simulink model "yalinySatSim"  (R2015b)
settings: Solver=ode45  StartTime=0.0  StopTime=100  RelTol=1e-3
values from neighbouring files (symbols this model uses):
  orbData =     [orbitData.mat]
undefined symbols (not defined in the file or in its folder): e0_0, e1_0, e2_0, e3_0, params
libraries: aerolibutil x16, vrlib x16, satellite_control_lib x11, aerolibtransform2 x3, aerolib6dofsys x2, simulink_extras x1
settings Model: Creator=DNikolaev  LastModifiedBy=DNikolaev

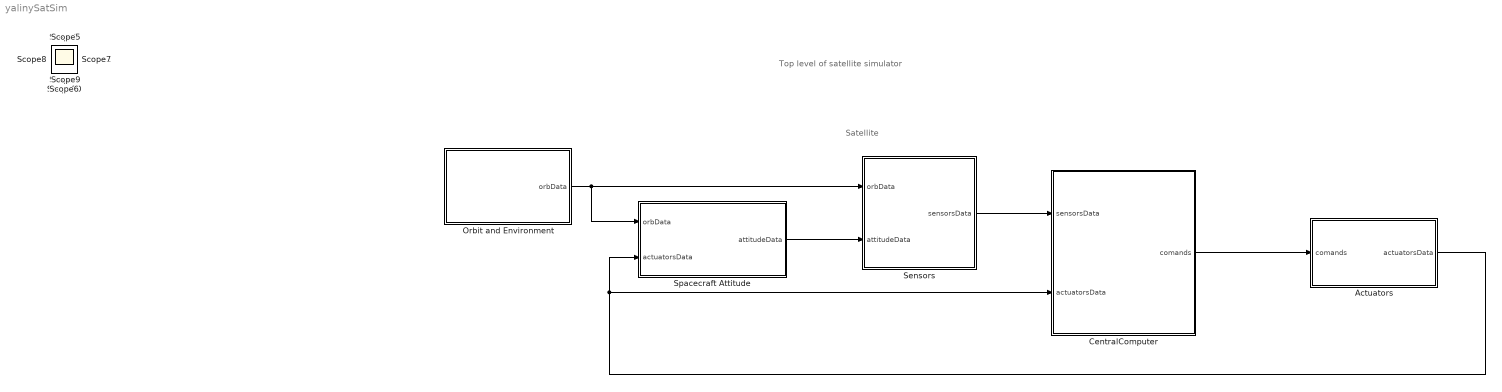
== system yalinySatSim ==
  note: Satellite
  note: Top level of satellite simulator
  Actuators : Subsystem
  CentralComputer : Subsystem
  Orbit and Environment : Subsystem
  Sensors : Subsystem
  Spacecraft Attitude : Subsystem
  Scope{,1..10} (11 alike) : Scope
  wires:
  Sensors/1(sensorsData) -> CentralComputer/1(sensorsData)
  Actuators/1(actuatorsData) -> CentralComputer/2(actuatorsData), Spacecraft Attitude/2(actuatorsData)
  CentralComputer/1(comands) -> Actuators/1(comands)
  Orbit and Environment/1(orbData) -> Spacecraft Attitude/1(orbData), Sensors/1(orbData)
  Spacecraft Attitude/1(attitudeData) -> Sensors/2(attitudeData)

== system yalinySatSim/Actuators ==
  comands : Inport
  Bus Creator : BusCreator  Inputs=3
  Bus Selector4 : BusSelector  OutputSignals=Urw,Umagn
  Constant2 : Constant  Value=[0 0 0]
  Magnetic Coils : satellite_control_lib/Actuators/Magnetic Coils  MagnMomentMax=params.MagnMomentMax
  Manual Switch : ManualSwitch
  Reaction Wheels 4-pyramid configuration : satellite_control_lib/Actuators/Reaction Wheels 4-pyramid configuration  VariantControl=Variant  Hrwmax=params.Hrwmax  Trwmax=params.Trwmax  delta=params.rwdelta  gamma=params.rwgamma  sampleTime=0.1
  actuatorsData : Outport
  wires:
  comands/1 -> Bus Selector4/1
  Bus Creator/1 -> actuatorsData/1
  Magnetic Coils/1 -> Bus Creator/3  "L"
  Bus Selector4/1 -> Manual Switch/1  "<Urw>"
  Manual Switch/1 -> Reaction Wheels 4-pyramid configuration/1
  Constant2/1 -> Manual Switch/2
  Reaction Wheels 4-pyramid configuration/1 -> Bus Creator/1  "Trw_p"
  Reaction Wheels 4-pyramid configuration/2 -> Bus Creator/2  "Hrw_p"
  Bus Selector4/2 -> Magnetic Coils/1  "<Umagn >"

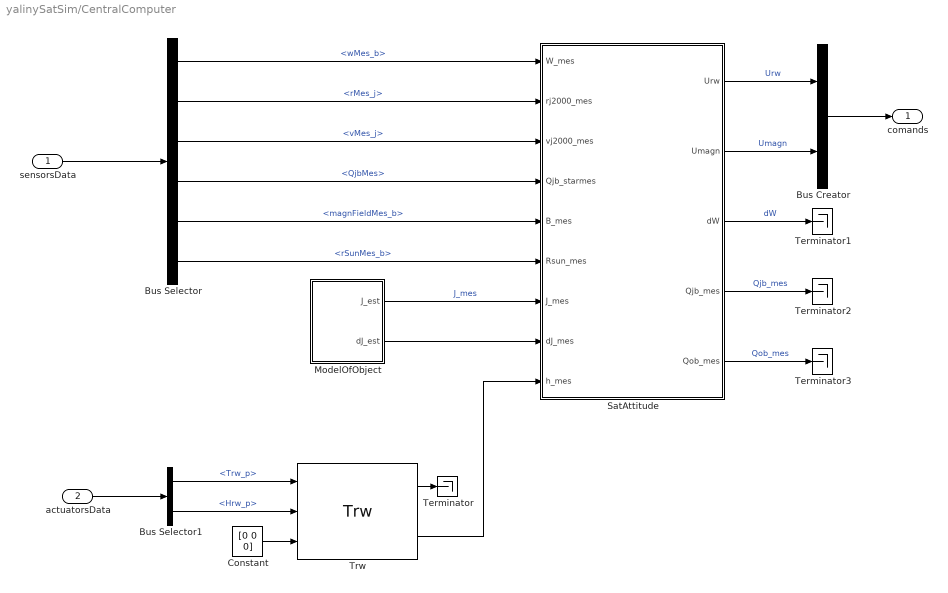
== system yalinySatSim/CentralComputer ==
  sensorsData : Inport
  actuatorsData : Inport  Port=2
  Bus Creator : BusCreator  Inputs=2
  Bus Selector : BusSelector  OutputSignals=wMes_b,rMes_j,vMes_j,QjbMes,magnFieldMes_b,rSunMes_b
  Bus Selector1 : BusSelector  OutputSignals=Trw_p,Hrw_p
  Constant : Constant  Value=[0 0 0]
  ModelOfObject : Subsystem
  SatAttitude : Subsystem
  Terminator{,1..3} (4 alike) : Terminator
  Trw : satellite_control_lib/Torques/Trw  delta=params.rwdelta  gamma=params.rwgamma
  comands : Outport
  wires:
  sensorsData/1 -> Bus Selector/1
  Bus Creator/1 -> comands/1
  ModelOfObject/1(J_est) -> SatAttitude/7(J_mes)  "J_mes"
  SatAttitude/1(Urw) -> Bus Creator/1  "Urw"
  ModelOfObject/2(dJ_est) -> SatAttitude/8(dJ_mes)
  Trw/2 -> SatAttitude/9(h_mes)
  actuatorsData/1 -> Bus Selector1/1
  Bus Selector/2 -> SatAttitude/2(rj2000_mes)  "<rMes_j>"
  Bus Selector/3 -> SatAttitude/3(vj2000_mes)  "<vMes_j>"
  Bus Selector/6 -> SatAttitude/6(Rsun_mes)  "<rSunMes_b>"
  Bus Selector/5 -> SatAttitude/5(B_mes)  "<magnFieldMes_b>"
  Bus Selector/1 -> SatAttitude/1(W_mes)  "<wMes_b>"
  Bus Selector/4 -> SatAttitude/4(Qjb_starmes)  "<QjbMes>"
  Bus Selector1/1 -> Trw/1  "<Trw_p>"
  Bus Selector1/2 -> Trw/2  "<Hrw_p>"
  Trw/1 -> Terminator/1
  Constant/1 -> Trw/3
  SatAttitude/3(dW) -> Terminator1/1  "dW"
  SatAttitude/4(Qjb_mes) -> Terminator2/1  "Qjb_mes"
  SatAttitude/5(Qob_mes) -> Terminator3/1  "Qob_mes"
  SatAttitude/2("Umagn ") -> Bus Creator/2  "Umagn"

== system yalinySatSim/Orbit and Environment ==
  Precomputed Data : FromWorkspace  VariableName=inOrbData  OutDataTypeStr=Bus: orbBus  SampleTime=0  OutputAfterFinalValue=Holding final value
  orbData : Outport
  wires:
  Precomputed Data/1 -> orbData/1

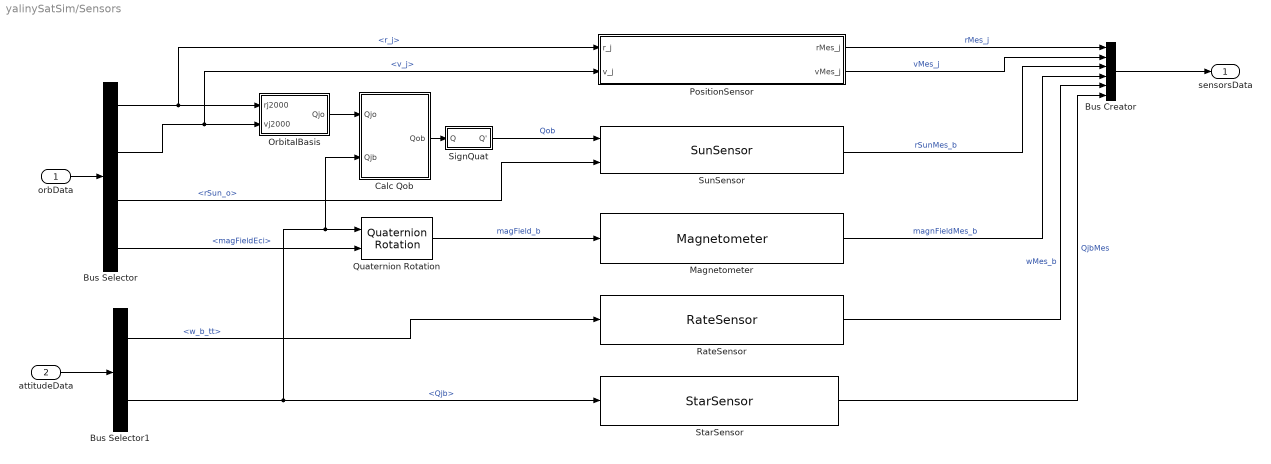
== system yalinySatSim/Sensors ==
  orbData : Inport
  attitudeData : Inport  Port=2
  Bus Creator : BusCreator  Inputs=6
  Bus Selector : BusSelector  OutputSignals=r_j,v_j,rSun_o,magFieldEci
  Bus Selector1 : BusSelector  OutputSignals=w_b_tt,Qjb
  Calc Qob : Subsystem
  Magnetometer : satellite_control_lib/Sensors/Magnetometer  S=[0 0 0;0 0 0;0 0 0]  bias=0  sigma2=0  seed=0  outputSampleTime=0.1
  OrbitalBasis : Subsystem
  PositionSensor : Subsystem
  Quaternion Rotation : aerolibutil/Quaternion Rotation
  RateSensor : satellite_control_lib/Sensors/RateSensor  S=[0 0 0;0 0 0;0 0 0]  sigma2_b=0  seed_b=[0 0 0]  sigma2_n=1e-6  seed=[0 0 0]  rateSensorSamleTime=0.1
  SignQuat : Subsystem
  StarSensor : satellite_control_lib/Sensors/StarSensor  sigma2=[0 0 0]  seed=[0 0 0]  outputSamleTime=0.1
  SunSensor : satellite_control_lib/Sensors/SunSensor  sigma2=[0 0 0]  seed=[0 0 0]  outputSampleTime=0.1
  sensorsData : Outport
  wires:
  orbData/1 -> Bus Selector/1
  attitudeData/1 -> Bus Selector1/1
  Bus Selector/1 -> PositionSensor/1(r_j), OrbitalBasis/1(rj2000)  "<r_j>"
  Bus Selector/2 -> PositionSensor/2(v_j), OrbitalBasis/2(vj2000)  "<v_j>"
  Bus Selector/3 -> SunSensor/2  "<rSun_o>"
  Bus Selector/4 -> Quaternion Rotation/2  "<magFieldEci>"
  Bus Selector1/2 -> Quaternion Rotation/1, Calc Qob/2(Qjb), StarSensor/1  "<Qjb>"
  Bus Selector1/1 -> RateSensor/1  "<w_b_tt>"
  Bus Creator/1 -> sensorsData/1
  RateSensor/1 -> Bus Creator/5  "wMes_b"
  Quaternion Rotation/1 -> Magnetometer/1  "magField_b"
  Magnetometer/1 -> Bus Creator/4  "magnFieldMes_b"
  Calc Qob/1(Qob) -> SignQuat/1(Q)
  OrbitalBasis/1(Qjo) -> Calc Qob/1(Qjo)
  SignQuat/1(Q') -> SunSensor/1  "Qob"
  SunSensor/1 -> Bus Creator/3  "rSunMes_b"
  PositionSensor/1(rMes_j) -> Bus Creator/1  "rMes_j"
  PositionSensor/2(vMes_j) -> Bus Creator/2  "vMes_j"
  StarSensor/1 -> Bus Creator/6  "QjbMes"

== system yalinySatSim/Spacecraft Attitude ==
  orbData : Inport
  actuatorsData : Inport  Port=2
  Bus Creator : BusCreator  Inputs=2
  Inertia : Subsystem
  Spacecraft Dynamics : Subsystem
  Torques : Subsystem
  attitudeData : Outport
  wires:
  Torques/1(T) -> Spacecraft Dynamics/1(T)
  Inertia/1(Inertia) -> Spacecraft Dynamics/2(Inertia), Torques/5(Inertia)
  Inertia/2(dInertia) -> Spacecraft Dynamics/3(dInertia)
  Spacecraft Dynamics/2(w_b) -> Bus Creator/2, Torques/2(w_b)  "w_b_tt"
  Bus Creator/1 -> attitudeData/1
  orbData/1 -> Torques/3(orbData)
  actuatorsData/1 -> Torques/4(actuatorsData)
  Spacecraft Dynamics/1(Qjb) -> Torques/1(Qjb), Bus Creator/1  "Qjb"

== system yalinySatSim/CentralComputer/ModelOfObject ==
  ChangeMe1 : Constant  Value=zeros(3)
  ChangeMe2 : Constant  Value=1000*eye(3)
  J_est : Outport
  dJ_est : Outport  Port=2
  wires:
  ChangeMe1/1 -> dJ_est/1
  ChangeMe2/1 -> J_est/1

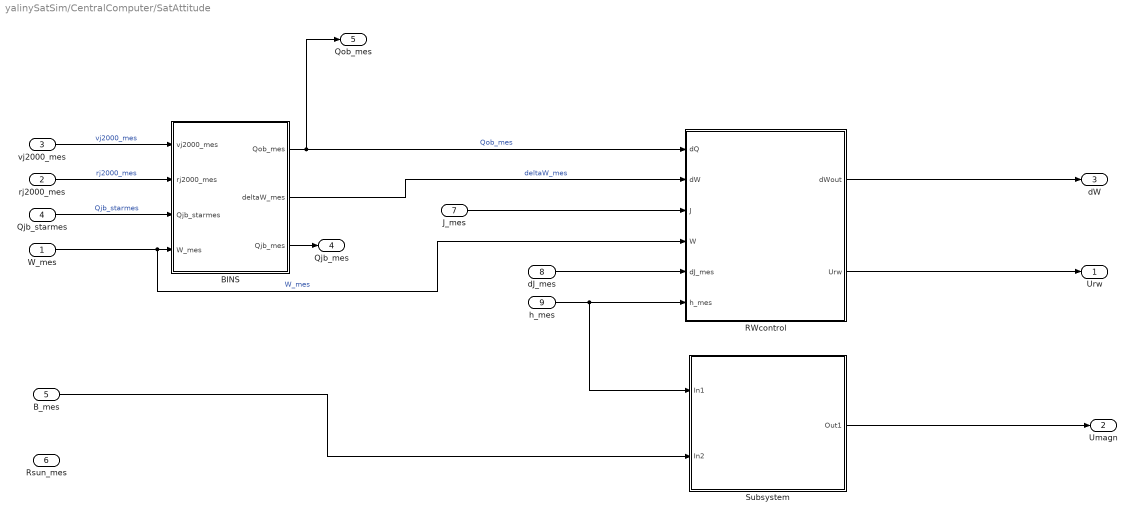
== system yalinySatSim/CentralComputer/SatAttitude ==
  W_mes : Inport
  rj2000_mes : Inport  Port=2
  vj2000_mes : Inport  Port=3
  Qjb_starmes : Inport  Port=4
  B_mes : Inport  Port=5
  Rsun_mes : Inport  Port=6
  J_mes : Inport  Port=7
  dJ_mes : Inport  Port=8
  h_mes : Inport  Port=9
  BINS : Subsystem
  RWcontrol : Subsystem
  Subsystem : Subsystem
  Urw : Outport
  "Umagn " : Outport  Port=2
  dW : Outport  Port=3
  Qjb_mes : Outport  Port=4
  Qob_mes : Outport  Port=5
  wires:
  vj2000_mes/1 -> BINS/1(vj2000_mes)  "vj2000_mes"
  rj2000_mes/1 -> BINS/2(rj2000_mes)  "rj2000_mes"
  Qjb_starmes/1 -> BINS/3(Qjb_starmes)  "Qjb_starmes"
  W_mes/1 -> RWcontrol/4(W), BINS/4(W_mes)  "W_mes"
  BINS/1(Qob_mes) -> Qob_mes/1, RWcontrol/1(dQ)  "Qob_mes"
  BINS/3(Qjb_mes) -> Qjb_mes/1
  BINS/2(deltaW_mes) -> RWcontrol/2(dW)  "deltaW_mes"
  J_mes/1 -> RWcontrol/3(J)
  dJ_mes/1 -> RWcontrol/5(dJ_mes)
  h_mes/1 -> Subsystem/1(In1), RWcontrol/6(h_mes)
  RWcontrol/1(dWout) -> dW/1
  RWcontrol/2(Urw) -> Urw/1
  B_mes/1 -> Subsystem/2(In2)
  Subsystem/1(Out1) -> "Umagn "/1

== system yalinySatSim/Sensors/Calc Qob ==
  Qjo : Inport
  Qjb : Inport  Port=2
  Quaternion Inverse : aerolibutil/Quaternion Inverse
  Quaternion Multiplication : aerolibutil/Quaternion Multiplication
  Qob : Outport
  wires:
  Qjb/1 -> Quaternion Multiplication/2  "Qjb"
  Qjo/1 -> Quaternion Inverse/1  "Qjo"
  Quaternion Inverse/1 -> Quaternion Multiplication/1
  Quaternion Multiplication/1 -> Qob/1

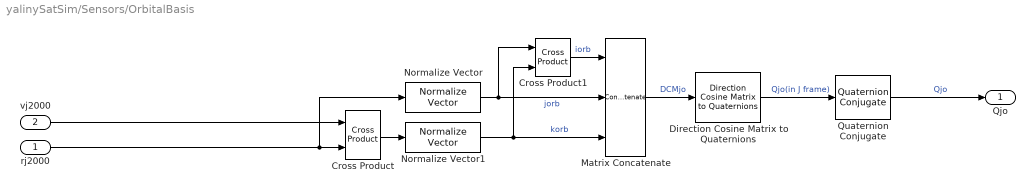
== system yalinySatSim/Sensors/OrbitalBasis ==
  rj2000 : Inport
  vj2000 : Inport  Port=2
  Cross Product : vrlib/Utilities/Cross Product
  Cross Product1 : vrlib/Utilities/Cross Product
  Direction Cosine Matrix to Quaternions : aerolibtransform2/Direction Cosine Matrix  to Quaternions
  Matrix Concatenate : Concatenate  NumInputs=3  Mode=Multidimensional array  ConcatenateDimension=2
  Normalize Vector : vrlib/Utilities/Normalize Vector  maxzero=0.00001
  Normalize Vector1 : vrlib/Utilities/Normalize Vector  maxzero=0.00001
  Quaternion Conjugate : aerolibutil/Quaternion Conjugate
  Qjo : Outport
  wires:
  Quaternion Conjugate/1 -> Qjo/1  "Qjo"
  Cross Product/1 -> Normalize Vector1/1
  Normalize Vector1/1 -> Cross Product1/2, Matrix Concatenate/3  "korb"
  Direction Cosine Matrix to Quaternions/1 -> Quaternion Conjugate/1  "Qjo(in J frame)"
  vj2000/1 -> Cross Product/1
  rj2000/1 -> Cross Product/2, Normalize Vector/1
  Matrix Concatenate/1 -> Direction Cosine Matrix to Quaternions/1  "DCMjo"
  Normalize Vector/1 -> Cross Product1/1, Matrix Concatenate/2  "jorb"
  Cross Product1/1 -> Matrix Concatenate/1  "iorb"

== system yalinySatSim/Sensors/PositionSensor ==
  r_j : Inport
  v_j : Inport  Port=2
  Zero-Order Hold : ZeroOrderHold  SampleTime=0.1
  Zero-Order Hold1 : ZeroOrderHold  SampleTime=0.1
  rMes_j : Outport
  vMes_j : Outport  Port=2
  wires:
  Zero-Order Hold/1 -> rMes_j/1
  Zero-Order Hold1/1 -> vMes_j/1
  r_j/1 -> Zero-Order Hold/1
  v_j/1 -> Zero-Order Hold1/1

== system yalinySatSim/Sensors/SignQuat ==
  Q : Inport
  Product : Product
  Selector2 : Selector  InputPortWidth=4  IndexOptions=Index vector (dialog)  Indices=[1]  OutputSizes=1
  Sign : Signum
  Q' : Outport
  wires:
  Q/1 -> Product/2, Selector2/1
  Product/1 -> Q'/1
  Sign/1 -> Product/1
  Selector2/1 -> Sign/1

== system yalinySatSim/Spacecraft Attitude/Inertia ==
  bodysAttitude : Inport
  Constant : Constant  Value=1000*eye(3)
  Constant1 : Constant  Value=zeros(3)
  Inertia : Outport
  dInertia : Outport  Port=2
  wires:
  Constant1/1 -> dInertia/1
  Constant/1 -> Inertia/1

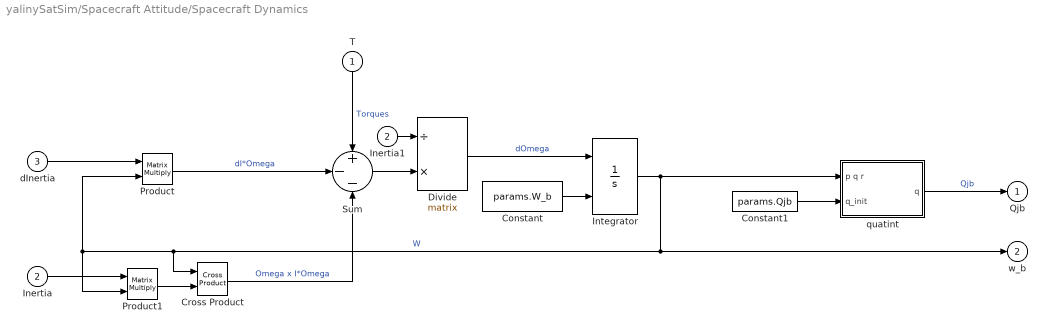
== system yalinySatSim/Spacecraft Attitude/Spacecraft Dynamics ==
  T : Inport
  Inertia : Inport  Port=2
  dInertia : Inport  Port=3
  Constant : Constant  Value=params.W_b
  Constant1 : Constant  Value=params.Qjb
  Cross Product : vrlib/Utilities/Cross Product
  Divide : Product  Inputs=/*  Multiplication=Matrix(*)
  Inertia1 : InportShadow  Port=2
  Integrator : Integrator  InitialConditionSource=external
  Product : Product  Multiplication=Matrix(*)
  Product1 : Product  Multiplication=Matrix(*)
  Sum : Sum  Inputs=+--
  quatint : Subsystem
  Qjb : Outport
  w_b : Outport  Port=2
  wires:
  Sum/1 -> Divide/2
  Inertia1/1 -> Divide/1
  Divide/1 -> Integrator/1  "dOmega"
  Constant/1 -> Integrator/2
  Product/1 -> Sum/2  "dI*Omega"
  dInertia/1 -> Product/1
  Constant1/1 -> quatint/2(q_init)
  quatint/1(q) -> Qjb/1  "Qjb"
  Inertia/1 -> Product1/1
  Product1/1 -> Cross Product/2
  Cross Product/1 -> Sum/3  "Omega x I*Omega"
  Integrator/1 -> quatint/1(p q r), Cross Product/1, Product/2, Product1/2, w_b/1  "W"
  T/1 -> Sum/1  "Torques"

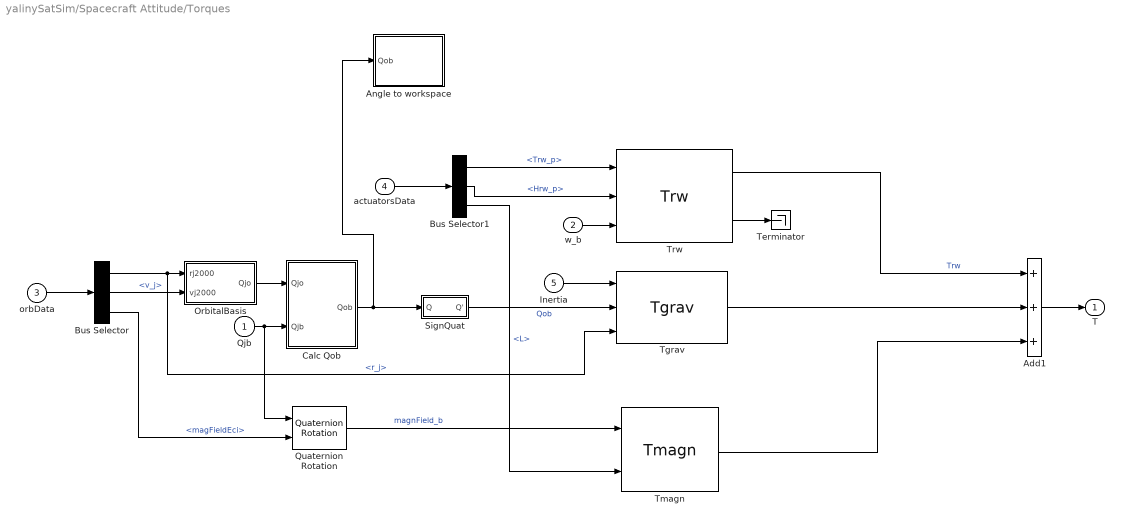
== system yalinySatSim/Spacecraft Attitude/Torques ==
  Qjb : Inport
  w_b : Inport  Port=2
  orbData : Inport  Port=3
  actuatorsData : Inport  Port=4
  Inertia : Inport  Port=5
  Add1 : Sum  Inputs=3
  Angle to workspace : Subsystem
  Bus Selector : BusSelector  OutputSignals=r_j,v_j,magFieldEci
  Bus Selector1 : BusSelector  OutputSignals=Trw_p,Hrw_p,L
  Calc Qob : Subsystem
  OrbitalBasis : Subsystem
  Quaternion Rotation : aerolibutil/Quaternion Rotation
  SignQuat : Subsystem
  Terminator : Terminator
  Tgrav : satellite_control_lib/Torques/Tgrav
  Tmagn : satellite_control_lib/Torques/Tmagn
  Trw : satellite_control_lib/Torques/Trw  delta=params.rwdelta  gamma=params.rwgamma
  T : Outport
  wires:
  Add1/1 -> T/1
  Trw/1 -> Add1/1  "Trw"
  Tgrav/1 -> Add1/2
  orbData/1 -> Bus Selector/1
  actuatorsData/1 -> Bus Selector1/1
  SignQuat/1(Q') -> Tgrav/2  "Qob"
  Bus Selector/1 -> Tgrav/3, OrbitalBasis/1(rj2000)  "<r_j>"
  Bus Selector/2 -> OrbitalBasis/2(vj2000)  "<v_j>"
  OrbitalBasis/1(Qjo) -> Calc Qob/1(Qjo)
  Qjb/1 -> Quaternion Rotation/1, Calc Qob/2(Qjb)
  Inertia/1 -> Tgrav/1
  w_b/1 -> Trw/3
  Bus Selector1/2 -> Trw/2  "<Hrw_p>"
  Bus Selector1/1 -> Trw/1  "<Trw_p>"
  Trw/2 -> Terminator/1
  Tmagn/1 -> Add1/3
  Bus Selector/3 -> Quaternion Rotation/2  "<magFieldEci>"
  Quaternion Rotation/1 -> Tmagn/1  "magnField_b"
  Bus Selector1/3 -> Tmagn/2  "<L>"
  Calc Qob/1(Qob) -> Angle to workspace/1(Qob), SignQuat/1(Q)

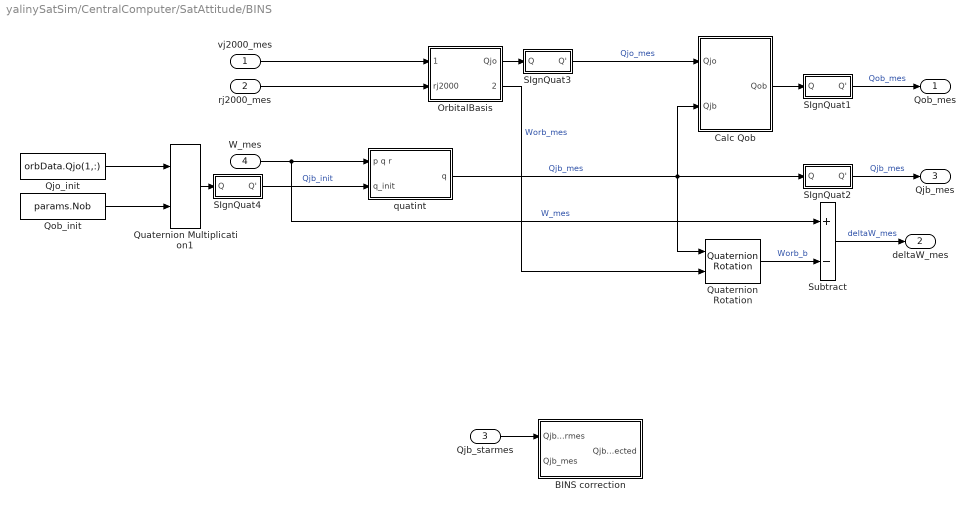
== system yalinySatSim/CentralComputer/SatAttitude/BINS ==
  vj2000_mes : Inport
  rj2000_mes : Inport  Port=2
  Qjb_starmes : Inport  Port=3
  W_mes : Inport  Port=4
  BINS correction : Subsystem
  Calc Qob : Subsystem
  OrbitalBasis : Subsystem
  Qjo_init : Constant  Value=orbData.Qjo(1,:)
  Qob_init : Constant  Value=params.Nob
  Quaternion Multiplication1 : aerolibutil/Quaternion Multiplication
  Quaternion Rotation : aerolibutil/Quaternion Rotation
  SIgnQuat1 : Subsystem
  SIgnQuat2 : Subsystem
  SIgnQuat3 : Subsystem
  SIgnQuat4 : Subsystem
  Subtract : Sum  Inputs=+-
  quatint : Subsystem  mask{k_quat=1}
      mask prompts: k_quat "Quaternion normalization gain"
  Qob_mes : Outport
  deltaW_mes : Outport  Port=2
  Qjb_mes : Outport  Port=3
  wires:
  Qjb_starmes/1 -> BINS correction/1(Qjb_starmes)
  quatint/1(q) -> SIgnQuat2/1(Q), Calc Qob/2(Qjb), Quaternion Rotation/1  "Qjb_mes"
  Calc Qob/1(Qob) -> SIgnQuat1/1(Q)
  rj2000_mes/1 -> OrbitalBasis/2(rj2000)
  vj2000_mes/1 -> OrbitalBasis/1(vj2000)
  OrbitalBasis/1(Qjo) -> SIgnQuat3/1(Q)
  OrbitalBasis/2(Worb_j) -> Quaternion Rotation/2  "Worb_mes"
  W_mes/1 -> Subtract/1, quatint/1(p q r)  "W_mes"
  Subtract/1 -> deltaW_mes/1  "deltaW_mes"
  Qjo_init/1 -> Quaternion Multiplication1/1
  Qob_init/1 -> Quaternion Multiplication1/2
  Quaternion Multiplication1/1 -> SIgnQuat4/1(Q)
  Quaternion Rotation/1 -> Subtract/2  "Worb_b"
  SIgnQuat1/1(Q') -> Qob_mes/1  "Qob_mes"
  SIgnQuat2/1(Q') -> Qjb_mes/1  "Qjb_mes"
  SIgnQuat3/1(Q') -> Calc Qob/1(Qjo)  "Qjo_mes"
  SIgnQuat4/1(Q') -> quatint/2(q_init)  "Qjb_init"

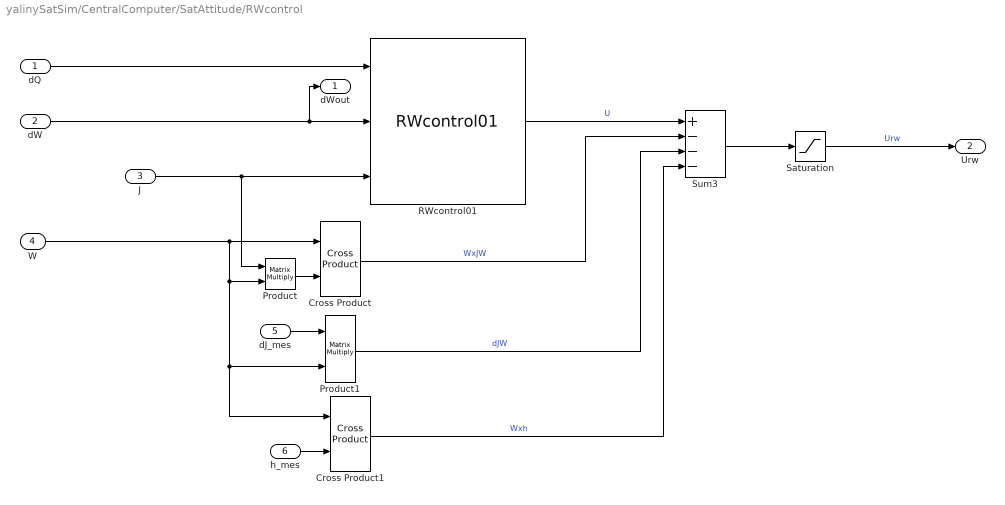
== system yalinySatSim/CentralComputer/SatAttitude/RWcontrol ==
  dQ : Inport
  dW : Inport  Port=2
  J : Inport  Port=3
  W : Inport  Port=4
  dJ_mes : Inport  Port=5
  h_mes : Inport  Port=6
  Cross Product : vrlib/Utilities/Cross Product
  Cross Product1 : vrlib/Utilities/Cross Product
  Product : Product  Multiplication=Matrix(*)
  Product1 : Product  Multiplication=Matrix(*)
  RWcontrol01 : satellite_control_lib/RWcontrol01  Kq=params.K1acs  Kw=params.K2acs
  Saturation : Saturate  UpperLimit=0.1  LowerLimit=-0.1
  Sum3 : Sum  Inputs=+---
  dWout : Outport
  Urw : Outport  Port=2
  wires:
  W/1 -> Product/2, Product1/2, Cross Product1/1, Cross Product/1
  dQ/1 -> RWcontrol01/1
  RWcontrol01/1 -> Sum3/1  "U"
  J/1 -> Product/1, RWcontrol01/3
  dW/1 -> dWout/1, RWcontrol01/2
  Product/1 -> Cross Product/2
  Cross Product/1 -> Sum3/2  "WxJW"
  Product1/1 -> Sum3/3  "dJW"
  Cross Product1/1 -> Sum3/4  "Wxh"
  h_mes/1 -> Cross Product1/2
  dJ_mes/1 -> Product1/1
  Saturation/1 -> Urw/1  "Urw"
  Sum3/1 -> Saturation/1

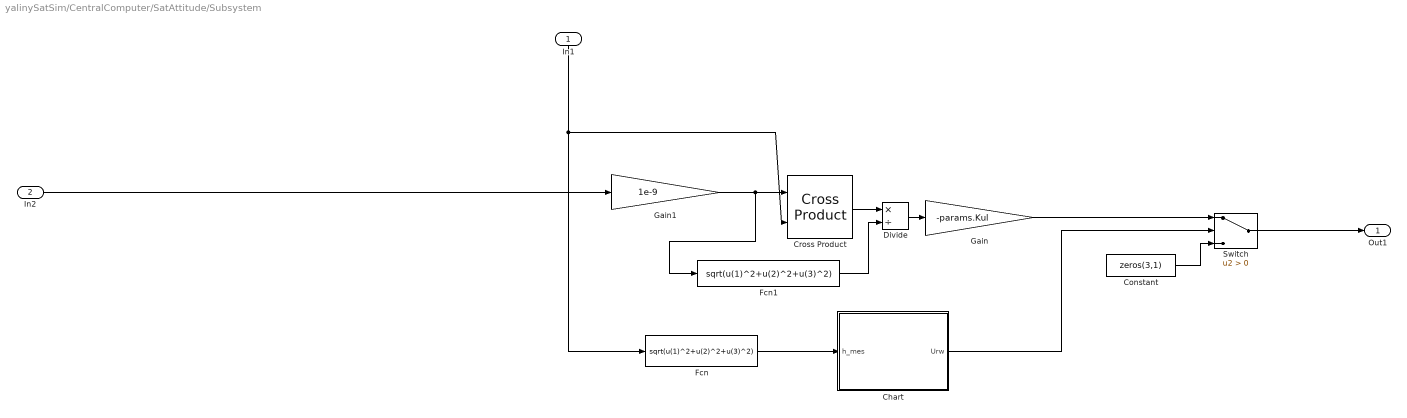
== system yalinySatSim/CentralComputer/SatAttitude/Subsystem ==
  In1 : Inport
  In2 : Inport  Port=2
  Chart : Stateflow chart  TreatAsAtomicUnit=on
  Constant : Constant  Value=zeros(3,1)
  Cross Product : vrlib/Utilities/Cross Product
  Divide : Product  Inputs=*/
  Fcn : Fcn  Expr=sqrt(u(1)^2+u(2)^2+u(3)^2)
  Fcn1 : Fcn  Expr=sqrt(u(1)^2+u(2)^2+u(3)^2)
  Gain : Gain  Gain=-params.Kul
  Gain1 : Gain  Gain=1e-9
  Switch : Switch  Criteria=u2 > Threshold
  Out1 : Outport
  wires:
  In1/1 -> Cross Product/2, Fcn/1
  In2/1 -> Gain1/1
  Gain1/1 -> Fcn1/1, Cross Product/1
  Divide/1 -> Gain/1
  Cross Product/1 -> Divide/1
  Fcn1/1 -> Divide/2
  Gain/1 -> Switch/1
  Fcn/1 -> Chart/1(h_mes)
  Chart/1(Urw) -> Switch/2
  Switch/1 -> Out1/1
  Constant/1 -> Switch/3

== system yalinySatSim/Spacecraft Attitude/Spacecraft Dynamics/quatint ==
  p q r : Inport
  q_init : Inport  Port=2
  q0 q1 q2 q3 : Integrator  InitialConditionSource=external  InitialCondition=[e0_0 e1_0 e2_0 e3_0]
  qdot : aerolib6dofsys/DCM & Euler Angles (Quaternion)/qdot
  q : Outport
  wires:
  q0 q1 q2 q3/1 -> q/1, qdot/2
  q_init/1 -> q0 q1 q2 q3/2
  p q r/1 -> qdot/1
  qdot/1 -> q0 q1 q2 q3/1

== system yalinySatSim/Spacecraft Attitude/Torques/Angle to workspace ==
  Qob : Inport
  Angle minuts : Gain  Gain=60
  Gain : Gain  Gain=2
  Product : Product
  Radians to Degrees : simulink_extras/Transformations/Radians to Degrees
  Selector : Selector  InputPortWidth=4  IndexOptions=Index vector (dialog)  Indices=[2 3 4]  OutputSizes=1
  Selector1 : Selector  InputPortWidth=4  IndexOptions=Index vector (dialog)  Indices=1  OutputSizes=1
  To Workspace : ToWorkspace  VariableName=qq  SaveFormat=Timeseries  SampleTime=-1
  wires:
  Product/1 -> Gain/1
  Selector1/1 -> Product/1
  Gain/1 -> Radians to Degrees/1
  Qob/1 -> Selector/1, Selector1/1
  Selector/1 -> Product/2
  Radians to Degrees/1 -> Angle minuts/1
  Angle minuts/1 -> To Workspace/1

== system yalinySatSim/Spacecraft Attitude/Torques/Calc Qob ==
  Qjo : Inport
  Qjb : Inport  Port=2
  Quaternion Inverse : aerolibutil/Quaternion Inverse
  Quaternion Multiplication : aerolibutil/Quaternion Multiplication
  Qob : Outport
  wires:
  Qjb/1 -> Quaternion Multiplication/2  "Qjb"
  Qjo/1 -> Quaternion Inverse/1  "Qjo"
  Quaternion Inverse/1 -> Quaternion Multiplication/1
  Quaternion Multiplication/1 -> Qob/1

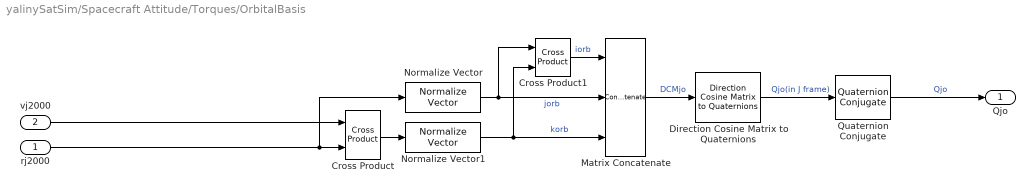
== system yalinySatSim/Spacecraft Attitude/Torques/OrbitalBasis ==
  rj2000 : Inport
  vj2000 : Inport  Port=2
  Cross Product : vrlib/Utilities/Cross Product
  Cross Product1 : vrlib/Utilities/Cross Product
  Direction Cosine Matrix to Quaternions : aerolibtransform2/Direction Cosine Matrix  to Quaternions
  Matrix Concatenate : Concatenate  NumInputs=3  Mode=Multidimensional array  ConcatenateDimension=2
  Normalize Vector : vrlib/Utilities/Normalize Vector  maxzero=0.00001
  Normalize Vector1 : vrlib/Utilities/Normalize Vector  maxzero=0.00001
  Quaternion Conjugate : aerolibutil/Quaternion Conjugate
  Qjo : Outport
  wires:
  Quaternion Conjugate/1 -> Qjo/1  "Qjo"
  Cross Product/1 -> Normalize Vector1/1
  Normalize Vector1/1 -> Cross Product1/2, Matrix Concatenate/3  "korb"
  Direction Cosine Matrix to Quaternions/1 -> Quaternion Conjugate/1  "Qjo(in J frame)"
  vj2000/1 -> Cross Product/1
  rj2000/1 -> Cross Product/2, Normalize Vector/1
  Matrix Concatenate/1 -> Direction Cosine Matrix to Quaternions/1  "DCMjo"
  Normalize Vector/1 -> Cross Product1/1, Matrix Concatenate/2  "jorb"
  Cross Product1/1 -> Matrix Concatenate/1  "iorb"

== system yalinySatSim/Spacecraft Attitude/Torques/SignQuat ==
  Q : Inport
  Product : Product
  Selector2 : Selector  InputPortWidth=4  IndexOptions=Index vector (dialog)  Indices=[1]  OutputSizes=1
  Sign : Signum
  Q' : Outport
  wires:
  Q/1 -> Product/2, Selector2/1
  Product/1 -> Q'/1
  Sign/1 -> Product/1
  Selector2/1 -> Sign/1

== system yalinySatSim/CentralComputer/SatAttitude/BINS/BINS correction ==
  Qjb_starmes : Inport
  Qjb_mes : Inport  Port=2
  Quaternion Conjugate : aerolibutil/Quaternion Conjugate
  Quaternion Conjugate1 : aerolibutil/Quaternion Conjugate
  Quaternion Multiplication : aerolibutil/Quaternion Multiplication
  Quaternion Multiplication1 : aerolibutil/Quaternion Multiplication
  Qjb_corrected : Outport
  wires:
  Quaternion Multiplication1/1 -> Qjb_corrected/1  "Qjb_corrected"
  Quaternion Conjugate1/1 -> Quaternion Multiplication1/1
  Qjb_mes/1 -> Quaternion Multiplication1/2, Quaternion Multiplication/2
  Quaternion Multiplication/1 -> Quaternion Conjugate1/1  "Nbb_mes"
  Qjb_starmes/1 -> Quaternion Conjugate/1
  Quaternion Conjugate/1 -> Quaternion Multiplication/1  "conjQjb_starmes"

== system yalinySatSim/CentralComputer/SatAttitude/BINS/Calc Qob ==
  Qjo : Inport
  Qjb : Inport  Port=2
  Quaternion Inverse : aerolibutil/Quaternion Inverse
  Quaternion Multiplication : aerolibutil/Quaternion Multiplication
  Qob : Outport
  wires:
  Qjb/1 -> Quaternion Multiplication/2  "Qjb"
  Qjo/1 -> Quaternion Inverse/1  "Qjo"
  Quaternion Inverse/1 -> Quaternion Multiplication/1
  Quaternion Multiplication/1 -> Qob/1

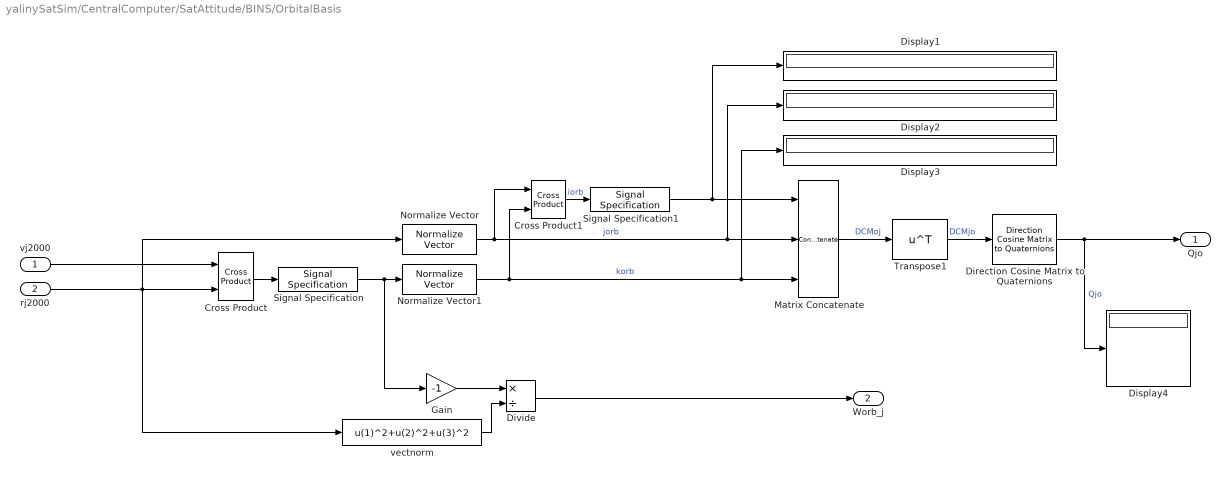
== system yalinySatSim/CentralComputer/SatAttitude/BINS/OrbitalBasis ==
  vj2000 : Inport
  rj2000 : Inport  Port=2
  Cross Product : vrlib/Utilities/Cross Product
  Cross Product1 : vrlib/Utilities/Cross Product
  Direction Cosine Matrix to Quaternions : aerolibtransform2/Direction Cosine Matrix  to Quaternions
  Display{1..4} (4 alike) : Display
  Divide : Product  Inputs=*/
  Gain : Gain  Gain=-1
  Matrix Concatenate : Concatenate  NumInputs=3  Mode=Multidimensional array  ConcatenateDimension=2
  Normalize Vector : vrlib/Utilities/Normalize Vector  maxzero=0.00001
  Normalize Vector1 : vrlib/Utilities/Normalize Vector  maxzero=0.00001
  Signal Specification : SignalSpecification  Dimensions=3
  Signal Specification1 : SignalSpecification  Dimensions=3
  Transpose1 : Math  Operator=transpose  SaturateOnIntegerOverflow=on
  vectnorm : Fcn  Expr=u(1)^2+u(2)^2+u(3)^2
  Qjo : Outport
  Worb_j : Outport  Port=2
  wires:
  Cross Product1/1 -> Signal Specification1/1  "iorb"
  Normalize Vector/1 -> Display2/1, Matrix Concatenate/2, Cross Product1/1  "jorb"
  Matrix Concatenate/1 -> Transpose1/1  "DCMoj"
  rj2000/1 -> Cross Product/2, Normalize Vector/1, vectnorm/1
  vj2000/1 -> Cross Product/1
  Direction Cosine Matrix to Quaternions/1 -> Display4/1, Qjo/1  "Qjo"
  Normalize Vector1/1 -> Display3/1, Matrix Concatenate/3, Cross Product1/2  "korb"
  Cross Product/1 -> Signal Specification/1
  Gain/1 -> Divide/1
  vectnorm/1 -> Divide/2
  Divide/1 -> Worb_j/1
  Signal Specification/1 -> Gain/1, Normalize Vector1/1
  Signal Specification1/1 -> Display1/1, Matrix Concatenate/1
  Transpose1/1 -> Direction Cosine Matrix to Quaternions/1  "DCMjo"

== system yalinySatSim/CentralComputer/SatAttitude/BINS/SIgnQuat1 ==
  Q : Inport
  Constant : Constant
  Constant1 : Constant  Value=-1
  Product : Product
  Selector2 : Selector  InputPortWidth=4  IndexOptions=Index vector (dialog)  Indices=[1]  OutputSizes=1
  Switch : Switch
  Q' : Outport
  wires:
  Q/1 -> Product/2, Selector2/1
  Product/1 -> Q'/1
  Switch/1 -> Product/1
  Selector2/1 -> Switch/2
  Constant/1 -> Switch/1
  Constant1/1 -> Switch/3

== system yalinySatSim/CentralComputer/SatAttitude/BINS/SIgnQuat2 ==
  Q : Inport
  Constant : Constant
  Constant1 : Constant  Value=-1
  Product : Product
  Selector2 : Selector  InputPortWidth=4  IndexOptions=Index vector (dialog)  Indices=[1]  OutputSizes=1
  Switch : Switch
  Q' : Outport
  wires:
  Q/1 -> Product/2, Selector2/1
  Product/1 -> Q'/1
  Switch/1 -> Product/1
  Selector2/1 -> Switch/2
  Constant/1 -> Switch/1
  Constant1/1 -> Switch/3

== system yalinySatSim/CentralComputer/SatAttitude/BINS/SIgnQuat3 ==
  Q : Inport
  Constant : Constant
  Constant1 : Constant  Value=-1
  Product : Product
  Selector2 : Selector  InputPortWidth=4  IndexOptions=Index vector (dialog)  Indices=[1]  OutputSizes=1
  Switch : Switch
  Q' : Outport
  wires:
  Q/1 -> Product/2, Selector2/1
  Product/1 -> Q'/1
  Switch/1 -> Product/1
  Selector2/1 -> Switch/2
  Constant/1 -> Switch/1
  Constant1/1 -> Switch/3

== system yalinySatSim/CentralComputer/SatAttitude/BINS/SIgnQuat4 ==
  Q : Inport
  Constant : Constant
  Constant1 : Constant  Value=-1
  Product : Product
  Selector2 : Selector  InputPortWidth=4  IndexOptions=Index vector (dialog)  Indices=[1]  OutputSizes=1
  Switch : Switch
  Q' : Outport
  wires:
  Q/1 -> Product/2, Selector2/1
  Product/1 -> Q'/1
  Switch/1 -> Product/1
  Selector2/1 -> Switch/2
  Constant/1 -> Switch/1
  Constant1/1 -> Switch/3

== system yalinySatSim/CentralComputer/SatAttitude/BINS/quatint ==
  p q r : Inport
  q_init : Inport  Port=2
  q0 q1 q2 q3 : Integrator  InitialConditionSource=external  InitialCondition=[e0_0 e1_0 e2_0 e3_0]
  qdot : aerolib6dofsys/DCM & Euler Angles (Quaternion)/qdot
  q : Outport
  wires:
  q0 q1 q2 q3/1 -> q/1, qdot/2
  q_init/1 -> q0 q1 q2 q3/2
  p q r/1 -> qdot/1
  qdot/1 -> q0 q1 q2 q3/1

== stateflow chart yalinySatSim/CentralComputer/SatAttitude/Subsystem/Chart ==
  state Whait
    entry:
    Urw=false;
  state Unload
    entry:
    Urw=true;
  (default) -> Whait
  Unload -> Whait : [h_mes < 0.1]
  Whait -> Unload : [h_mes > 1]
  data: h_mes input; Urw output
